simulink model "BDot32015a"  (R2015a)
settings: Solver=ode45  StartTime=0.01  StopTime=tprop  RelTol=1e-3
values from neighbouring files (symbols this model uses):
  epsilon0 = q(2:4)    [SetUp.m]
  eta0 = q(1)    [SetUp.m]
  euler0 = [Roll Pitch Yaw]'    [SetUp.m]
  hy = h(2)    [SetUp.m]
  J = [(1/12)*m*h^2 0 0 ; 0 (1/12)*m*h^2 0; 0 0 .5*m*r^2]    [SetUp.m]
  Jinv = inv(J)    [SetUp.m]
  kd = 100000000*J*2*zeta*nf    [SetUp.m]
  kdPoint = kd./[1 1 1; 1 10000000 1; 1 1 1]'    [SetUp.m]
  mu = 398600    [COES2rvd.m]    (also in SetUp.m; test.m)
  rvect = invconvmat*rvectx    [COES2rvd.m]    (also in test.m = rvect')
  T = 2*pi*sqrt(a^3/mu)    [SetUp.m]
  TcON = -1    [SetUp.m]
  Td = 0    [SetUp.m]
  tol = [.5e-5 .5e-5 .5e-5]    [SetUp.m]
  vvect = invconvmat*vvectx    [COES2rvd.m]    (also in test.m = vvect')
  wbn0 = DCM*w    [SetUp.m]
undefined symbols (not defined in the file or in its folder): IAU
libraries: aerolibtransform2 x2, simulink x1, aerolibgravity2 x1
settings Model: Creator=Trent  LastModifiedBy=morganyost

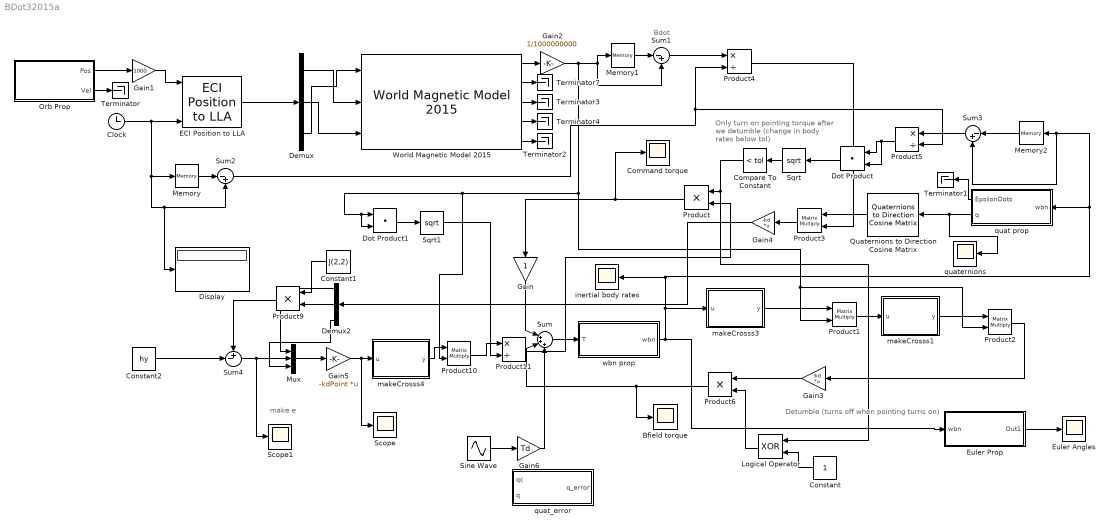
== system BDot32015a ==
  note: make e
  note: Detumble (turns off when pointing turns on)
  note: Only turn on pointing torque
      |  after we detumble
      | (change in body rates below tol)
  note: Bdot
  Bfield torque : Scope
      settings: TimeRange=auto  MaxDataPoints=5000  SaveToWorkspace=off  SaveName=ScopeData2  YMin=-0.000028  YMax=0.000058  SampleTime=-1
  Clock : Clock
  Command torque : Scope
      settings: TimeRange=auto  MaxDataPoints=5000  SaveToWorkspace=off  YMin=-0.0036  YMax=0.01275  SampleTime=-1
  Compare To Constant : simulink/Logic and Bit Operations/Compare To Constant  relop=<  const=tol  OutDataTypeStr=boolean  ZeroCross=off
  Constant : Constant
  Constant1 : Constant  Value=J(2,2)
  Constant2 : Constant  Value=hy
  Demux : Demux  Outputs=3
  Demux2 : Demux  Outputs=3
  Display : Display
  Dot Product : DotProduct  InputSameDT=on  OutDataTypeStr=Inherit: Inherit via internal rule
  Dot Product1 : DotProduct  InputSameDT=on  OutDataTypeStr=Inherit: Inherit via internal rule
  ECI Position to LLA : aerolibtransform2/ECI Position to LLA  red=IAU-2000/2006  year=2015  month=December  day=2  hour=0  min=0  sec=0  deltaT=Sec  errorflag=Error  extraparamflag=on  eunits=Metric (MKS)  earthmodel=WGS84  flat=1/298.257223563  eqradius=6378137
      settings: AttributesFormatString=%<red>
  Euler Angles : Scope
      settings: TimeRange=auto  ShowLegends=on  MaxDataPoints=5000  SaveToWorkspace=off  SaveName=ScopeData6  YMin=-46.16943  YMax=16.41945  SampleTime=-1
  Euler Prop : Subsystem  TreatAsAtomicUnit=on
  Gain : Gain
  Gain1 : Gain  Gain=1000
  Gain2 : Gain  Gain=1/1000000000
  Gain3 : Gain  Gain=-kd  Multiplication=Matrix(K*u)
  Gain4 : Gain  Gain=-kd  Multiplication=Matrix(K*u)
  Gain5 : Gain  Gain=-kdPoint  Multiplication=Matrix(K*u)
  Gain6 : Gain  Gain=Td
  Logical Operator : Logic  Operator=XOR  AllPortsSameDT=off  OutDataTypeStr=boolean
  Memory : Memory  X0=.0999999  InheritSampleTime=on
  Memory1 : Memory  X0=[2.1e-9;-5.8e-9;1e-9]  InheritSampleTime=on
  Memory2 : Memory  X0=wbn0+[.001;.001;.001]  InheritSampleTime=on
  Mux : Mux  Inputs=3
  Orb Prop : Subsystem
  Product : Product
  Product{1..3,10} (4 alike) : Product  Multiplication=Matrix(*)
  Product11 : Product  Inputs=*/
  Product4 : Product  Inputs=*/
  Product5 : Product  Inputs=*/
  Product6 : Product
  Product9 : Product
  Quaternions to Direction Cosine Matrix : aerolibtransform2/Quaternions to  Direction Cosine Matrix
  Scope : Scope
      settings: TimeRange=auto  MaxDataPoints=5000  SaveToWorkspace=off  SaveName=ScopeData4  YMin=-21911.297  YMax=197201.67302  SampleTime=-1
  Scope1 : Scope
      settings: TimeRange=auto  MaxDataPoints=5000  SaveToWorkspace=off  SaveName=ScopeData7  YMin=49632.44818  YMax=49636.58729  SampleTime=-1
  Sine Wave : Sin  Amplitude=1e-8  Frequency=100/T  SampleTime=0
  Sqrt : Sqrt  SaturateOnIntegerOverflow=on
  Sqrt1 : Sqrt  SaturateOnIntegerOverflow=on
  Sum : Sum  Inputs=|+++
  Sum1 : Sum  Inputs=|-+
  Sum2 : Sum  Inputs=|-+
  Sum3 : Sum  Inputs=|-+
  Sum4 : Sum  Inputs=+-|
  Terminator{,1..4,7} (6 alike) : Terminator
  World Magnetic Model 2015 : aerolibgravity2/World Magnetic Model 2015  RequirementInfo="{}  %GIDa_c707c699_7679_46e8_b9d9_c8e087eee6a8"  units=Metric (MKS)  time_in=off  month=December  day=2  year=2015  action=Error  h_out=on  dec_out=on  inc_out=on  ti_out=on
  inertial body rates : Scope
      settings: TimeRange=auto  ShowLegends=on  MaxDataPoints=5000  SaveToWorkspace=off  YMin=-0.09841  YMax=0.04872  SampleTime=-1
  makeCrosss1 : MATLAB Function  TreatAsAtomicUnit=on
      settings: PermitHierarchicalResolution=ParametersOnly
  makeCrosss3 : MATLAB Function  TreatAsAtomicUnit=on
      settings: PermitHierarchicalResolution=ParametersOnly
  makeCrosss4 : MATLAB Function  TreatAsAtomicUnit=on
      settings: PermitHierarchicalResolution=ParametersOnly
  quat prop : Subsystem
  quat_error : Subsystem
  quaternions : Scope
      settings: TimeRange=auto  ShowLegends=on  MaxDataPoints=5000  SaveToWorkspace=off  SaveName=ScopeData3  YMin=-1.22706  YMax=1.22156  SampleTime=-1
  wbn prop : Subsystem
  wires:
  ECI Position to LLA/1 -> Demux/1
  Clock/1 -> Memory/1, Display/1, Sum2/2, ECI Position to LLA/6
  Orb Prop/2(Vel) -> Terminator/1
  Demux/1 -> World Magnetic Model 2015/2
  Demux/2 -> World Magnetic Model 2015/3
  Demux/3 -> World Magnetic Model 2015/1
  Orb Prop/1(Pos) -> Gain1/1
  Gain1/1 -> ECI Position to LLA/1
  quat prop/2(q) -> quaternions/1, Quaternions to Direction Cosine Matrix/1
  quat prop/1(EpsilonDots) -> Terminator1/1
  Quaternions to Direction Cosine Matrix/1 -> Product3/1
  Memory/1 -> Sum2/1
  Memory1/1 -> Sum1/1
  World Magnetic Model 2015/1 -> Gain2/1
  makeCrosss3/1(y) -> Product1/1
  Product1/1 -> makeCrosss1/1(u)
  makeCrosss1/1(y) -> Product2/1
  Product2/1 -> Gain3/1
  Compare To Constant/1 -> Logical Operator/1, Product/1
  Product3/1 -> Gain4/1
  Sum/1 -> wbn prop/1(T)
  Memory2/1 -> Sum3/1
  Sum1/1 -> Product4/1
  Sum2/1 -> Product5/2, Product4/2
  Product4/1 -> Product3/2
  Sum3/1 -> Product5/1
  Product5/1 -> Dot Product/2, Dot Product/1
  Product/1 -> Gain/1, Command torque/1
  Dot Product/1 -> Sqrt/1
  Sqrt/1 -> Compare To Constant/1
  World Magnetic Model 2015/5 -> Terminator2/1
  World Magnetic Model 2015/4 -> Terminator4/1
  World Magnetic Model 2015/3 -> Terminator3/1
  Product6/1 -> Sum/2, Bfield torque/1
  Constant/1 -> Logical Operator/2
  Gain3/1 -> Product6/1
  Logical Operator/1 -> Product6/2
  Gain/1 -> Sum/1
  wbn prop/1(wbn) -> Euler Prop/1(wbn), makeCrosss3/1(u), Sum3/2, Memory2/1, quat prop/1(wbn), inertial body rates/1
  Demux2/1 -> Mux/1
  Demux2/3 -> Mux/3
  Product9/1 -> Sum4/1
  Sum4/1 -> Scope1/1, Mux/2
  Demux2/2 -> Product9/2
  Constant1/1 -> Product9/1
  Mux/1 -> Gain5/1
  Gain5/1 -> Scope/1, makeCrosss4/1(u)
  World Magnetic Model 2015/2 -> Terminator7/1
  makeCrosss4/1(y) -> Product10/1
  Dot Product1/1 -> Sqrt1/1
  Product10/1 -> Product11/1
  Sqrt1/1 -> Product11/2
  Gain2/1 -> Dot Product1/2, Dot Product1/1, Product10/2, Product2/2, Product1/2, Memory1/1, Sum1/2
  Product11/1 -> Product/2
  Sine Wave/1 -> Gain6/1
  Euler Prop/1(Out1) -> Euler Angles/1
  Constant2/1 -> Sum4/2
  Gain6/1 -> Sum/3
  Gain4/1 -> Demux2/1

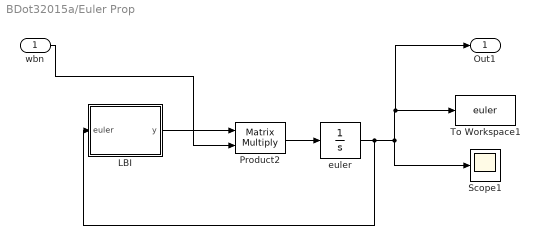
== system BDot32015a/Euler Prop ==
  wbn : Inport
  "LBI " : MATLAB Function  TreatAsAtomicUnit=on
      settings: PermitHierarchicalResolution=ParametersOnly
  Product2 : Product  Multiplication=Matrix(*)
  Scope1 : Scope
      settings: TimeRange=auto  LimitDataPoints=on  MaxDataPoints=5000  SaveToWorkspace=off  SaveName=ScopeData5  YMin=-10  YMax=10  SampleTime=-1  DataFormat=Array
  To Workspace1 : ToWorkspace  VariableName=euler  SaveFormat=Timeseries  SampleTime=-1
  euler : Integrator  InitialCondition=euler0
  Out1 : Outport
  wires:
  "LBI "/1(y) -> Product2/1
  Product2/1 -> euler/1
  euler/1 -> "LBI "/1(euler), Out1/1, To Workspace1/1, Scope1/1
  wbn/1 -> Product2/2

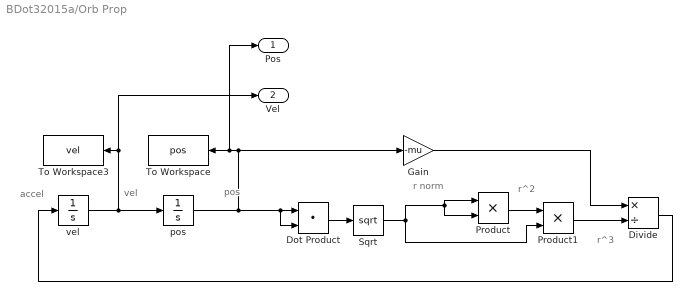
== system BDot32015a/Orb Prop ==
  note: r^3
  note: r^2
  note: r norm
  note: pos
  note: vel
  note: accel
  Divide : Product  Inputs=*/
  Dot Product : DotProduct  InputSameDT=on  OutDataTypeStr=Inherit: Inherit via internal rule
  Gain : Gain  Gain=-mu
  Product : Product
  Product1 : Product
  Sqrt : Sqrt  SaturateOnIntegerOverflow=on
  To Workspace : ToWorkspace  VariableName=pos  SaveFormat=Timeseries  SampleTime=-1
  To Workspace3 : ToWorkspace  VariableName=vel  SaveFormat=Timeseries  SampleTime=-1
  pos : Integrator  InitialCondition=rvect
  vel : Integrator  InitialCondition=vvect
  Pos : Outport
  Vel : Outport  Port=2
  wires:
  Sqrt/1 -> Product/2, Product/1, Product1/2
  Product/1 -> Product1/1
  Product1/1 -> Divide/2
  Gain/1 -> Divide/1
  Divide/1 -> vel/1
  Dot Product/1 -> Sqrt/1
  vel/1 -> Vel/1, To Workspace3/1, pos/1
  pos/1 -> Gain/1, Pos/1, To Workspace/1, Dot Product/2, Dot Product/1

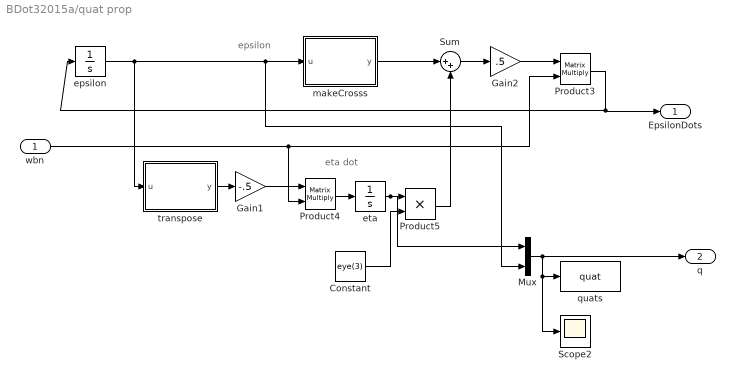
== system BDot32015a/quat prop ==
  note: eta dot
  note: epsilon
  wbn : Inport
  Constant : Constant  Value=eye(3)
  Gain1 : Gain  Gain=-.5
  Gain2 : Gain  Gain=.5
  Mux : Mux  Inputs=2
  Product3 : Product  Multiplication=Matrix(*)
  Product4 : Product  Multiplication=Matrix(*)
  Product5 : Product
  Scope2 : Scope
      settings: TimeRange=auto  LimitDataPoints=on  MaxDataPoints=5000  SaveToWorkspace=off  YMin=-10  YMax=10  SampleTime=-1  DataFormat=Array
  Sum : Sum  Inputs=|++
  epsilon : Integrator  InitialCondition=epsilon0
  eta : Integrator  InitialCondition=eta0
  makeCrosss : MATLAB Function  TreatAsAtomicUnit=on
      settings: PermitHierarchicalResolution=ParametersOnly
  quats : ToWorkspace  VariableName=quat  SaveFormat=Timeseries  SampleTime=-1
  transpose : MATLAB Function  TreatAsAtomicUnit=on
      settings: PermitHierarchicalResolution=ParametersOnly
  EpsilonDots : Outport
  q : Outport  Port=2
  wires:
  epsilon/1 -> Mux/2, makeCrosss/1(u), transpose/1(u)
  makeCrosss/1(y) -> Sum/1
  eta/1 -> Mux/1, Product5/1
  Product5/1 -> Sum/2
  Sum/1 -> Gain2/1
  Gain2/1 -> Product3/1
  Product3/1 -> EpsilonDots/1, epsilon/1
  Product4/1 -> eta/1
  transpose/1(y) -> Gain1/1
  Constant/1 -> Product5/2
  Gain1/1 -> Product4/1
  Mux/1 -> q/1, quats/1, Scope2/1
  wbn/1 -> Product3/2, Product4/2

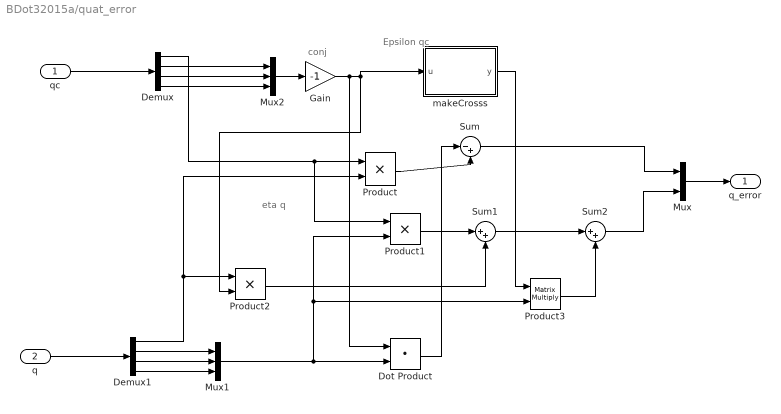
== system BDot32015a/quat_error ==
  note: conj
  note: eta q
  note: Epsilon qc
  qc : Inport
  q : Inport  Port=2
  Demux : Demux
  Demux1 : Demux
  Dot Product : DotProduct  InputSameDT=on  OutDataTypeStr=Inherit: Inherit via internal rule
  Gain : Gain  Gain=-1
  Mux : Mux  Inputs=2
  Mux1 : Mux  Inputs=3
  Mux2 : Mux  Inputs=3
  Product : Product
  Product1 : Product
  Product2 : Product
  Product3 : Product  Multiplication=Matrix(*)
  Sum : Sum  Inputs=|-+
  Sum1 : Sum  Inputs=|++
  Sum2 : Sum  Inputs=|++
  makeCrosss : MATLAB Function  TreatAsAtomicUnit=on
      settings: PermitHierarchicalResolution=ParametersOnly
  q_error : Outport
  wires:
  qc/1 -> Demux/1
  q/1 -> Demux1/1
  Demux/1 -> Product/1, Product1/1
  Demux1/1 -> Product/2, Product2/1
  Product/1 -> Sum/2
  Demux/2 -> Mux2/1
  Demux/3 -> Mux2/2
  Demux/4 -> Mux2/3
  Demux1/2 -> Mux1/1
  Demux1/3 -> Mux1/2
  Demux1/4 -> Mux1/3
  Mux2/1 -> Gain/1
  Dot Product/1 -> Sum/1
  Sum/1 -> Mux/1
  Product1/1 -> Sum1/1
  Product2/1 -> Sum1/2
  Sum1/1 -> Sum2/1
  Product3/1 -> Sum2/2
  makeCrosss/1(y) -> Product3/1
  Mux1/1 -> Product1/2, Product3/2, Dot Product/2
  Sum2/1 -> Mux/2
  Mux/1 -> q_error/1
  Gain/1 -> makeCrosss/1(u), Product2/2, Dot Product/1

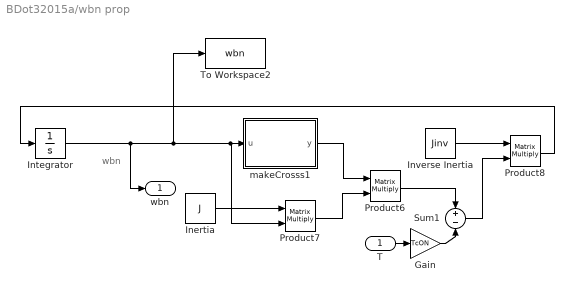
== system BDot32015a/wbn prop ==
  note: wbn
  T : Inport
  Gain : Gain  Gain=TcON
  Inertia : Constant  Value=J
  Integrator : Integrator  InitialCondition=wbn0
  Inverse Inertia : Constant  Value=Jinv
  Product6 : Product  Multiplication=Matrix(*)
  Product7 : Product  Multiplication=Matrix(*)
  Product8 : Product  Multiplication=Matrix(*)
  Sum1 : Sum  Inputs=+-
  To Workspace2 : ToWorkspace  VariableName=wbn  SaveFormat=Timeseries  SampleTime=-1
  makeCrosss1 : MATLAB Function  TreatAsAtomicUnit=on
      settings: PermitHierarchicalResolution=ParametersOnly
  wbn : Outport
  wires:
  makeCrosss1/1(y) -> Product6/1
  Inertia/1 -> Product7/1
  Product7/1 -> Product6/2
  Inverse Inertia/1 -> Product8/1
  Product8/1 -> Integrator/1
  Product6/1 -> Sum1/1
  Sum1/1 -> Product8/2
  Integrator/1 -> wbn/1, Product7/2, makeCrosss1/1(u), To Workspace2/1
  T/1 -> Gain/1
  Gain/1 -> Sum1/2

== matlab function BDot32015a/makeCrosss1 ==
  data: u input; y output
function y = fcn(u)
%#codegen
Ex = u(1);
Ey = u(2);
Ez = u(3);

y = [0 -Ez Ey; Ez 0 -Ex; -Ey Ex 0];

== matlab function BDot32015a/quat_error/makeCrosss ==
  data: u input; y output
function y = fcn(u)
%#codegen
Ex = u(1);
Ey = u(2);
Ez = u(3);

y = [0 -Ez Ey; Ez 0 -Ex; -Ey Ex 0];

== matlab function BDot32015a/quat prop/makeCrosss ==
  data: u input; y output
function y = fcn(u)
%#codegen
Ex = u(1);
Ey = u(2);
Ez = u(3);

y = [0 -Ez Ey; Ez 0 -Ex; -Ey Ex 0];

== matlab function BDot32015a/wbn prop/makeCrosss1 ==
  data: u input; y output
function y = fcn(u)
%#codegen
Ex = u(1);
Ey = u(2);
Ez = u(3);

y = [0 -Ez Ey; Ez 0 -Ex; -Ey Ex 0];

== matlab function BDot32015a/quat prop/transpose ==
  data: u input; y output
function y = fcn(u)
%#codegen

y = u';

== matlab function BDot32015a/makeCrosss4 ==
  data: u input; y output
function y = fcn(u)
%#codegen
Ex = u(1);
Ey = u(2);
Ez = u(3);

y = [0 -Ez Ey; Ez 0 -Ex; -Ey Ex 0];

== matlab function BDot32015a/makeCrosss3 ==
  data: u input; y output
function y = fcn(u)
%#codegen
Ex = u(1);
Ey = u(2);
Ez = u(3);

y = [0 -Ez Ey; Ez 0 -Ex; -Ey Ex 0];

== matlab function BDot32015a/Euler Prop/LBI  ==
  data: euler input; y output
function y = fcn(euler)
%#codegen
phi = euler(1);
theta = euler(2);
y = LBI(theta, phi);
